simulink model "RightInvariant_EKF"  (R2016b)
settings: Solver=FixedStepDiscrete  StartTime=0.0  StopTime=inf  RelTol=1e-3  EnableMultiTasking=on
InitFcn:
  | realTimeInitFcn;
  | StateEst_ini
undefined symbols (not defined in the file or in its folder): CassieParameters
libraries: StateEstimation_lib x1
settings Model: SimulationMode=external  TunableVars=B2_lpf_velocity_IMU,c_Kd,c_Kd_abduction,c_Kd_abduction_stand,c_Kd_knee,c_Kd_lateral_stand,c_Kd_pitch,c_Kd_roll,c_Kd_rotation,c_Kd_thigh,c_Kd_toe,c_Kd_toe_stand,c_Kfl_d,c_Kfl_p,c_Kfs_d,c_Kfs_p,c_Kp,c_Kp_abduction,c_Kp_abduction_stand,c_Kp_knee,c_Kp_lateral_stand,c_Kp_pitch,c_Kp_roll,c_Kp_rotation,c_Kp_thigh,c_Kp_toe,c_Kp_toe_stand,c_Kt_d,c_abduction_inward_gain,c_damping_gain,c_damping_threshold,c_fil_para,c_fil_para_x,c_fil_para_y,c_final_abduction,c_final_st_abduction,c_final_sw_LL_ext,c_final_sw_abduction,c_h_LL_cp,c_joint_filter_choice,c_lateral_offset,c_lateral_offset_default,c_lateral_velocity_weight,c_pre_final_sw_abduction,c_sagittal_offset,c_sagittal_offset_default,c_shift_distance,c_shift_time,c_stance_thre_lb,c_stance_thre_ub,c_stand_offset_default,c_standing_switch_time,c_test_frequency,c_test_joint,c_toe_tilt_angle,c_use_calib_spring,c_velocity_toe_tune  TunableVarsStorageClass=Auto,Auto,Auto,Auto,Auto,Auto,Auto,Auto,Auto,Auto,Auto,Auto,Auto,Auto,Auto,Auto,Auto,Auto,Auto,Auto,Auto,Auto,Auto,Auto,Auto,Auto,Auto,Auto,Auto,Auto,Auto,Auto,Auto,Auto,Auto,Auto,Auto,Auto,Auto,Auto,Auto,Auto,Auto,Auto,Auto,Auto,Auto,Auto,Auto,Auto,Auto,Auto,Auto,Auto,Auto,Auto,Auto  TunableVarsTypeQualifier=,,,,,,,,,,,,,,,,,,,,,,,,,,,,,,,,,,,,,,,,,,,,,,,,,,,,,,,,  Creator=robot  LastModifiedBy=Ross Hartley
settings SolverCC: EnableConcurrentExecution=on  ConcurrentTasks=on
settings DataIOCC: SaveFormat=Array  SaveOutput=off  SignalLogging=off  DSMLogging=off  VisualizeSimOutput=off  SaveTime=off
settings OptimizationCC: OptimizeBlockIOStorage=off  BufferReuse=off  GlobalBufferReuse=off  ExpressionFolding=off  LocalBlockOutputs=off  LifeSpan=inf  SimCompilerOptimization=on  AccelVerboseBuild=on
settings DebuggingCC: AllowSymbolicDim=off  SFUnexpectedBacktrackingDiag=warning  SFNoUnconditionalDefaultTransitionDiag=warning  SFExecutionAtInitializationDiag=none
settings HardwareCC: ProdBitPerPointer=32  ProdBitPerSizeT=32  ProdBitPerPtrDiffT=32  ProdLargestAtomicFloat=None  ProdWordSize=32  ProdLongLongMode=on  ProdHWDeviceType=Generic->32-bit x86 compatible
settings ModelReferenceCC: EnableParallelModelReferenceBuilds=on  ParallelModelReferenceMATLABWorkerInit=Copy Base Workspace  ModelReferenceNumInstancesAllowed=Single  PropagateSignalLabelsOutOfModel=off
settings SFSimCC: SFSimEcho=off
settings SFSimCC: SimUserSources=|
  | p_RightToeBottom_src.c
  | p_LeftToeBottom_src.c
  | J_RightToeBottom_src.c
  | J_LeftToeBottom_src.c
  | p_VectorNav_to_RightToeBottom_src.c
  | p_VectorNav_to_LeftToeBottom_src.c
  | J_VectorNav_to_RightToeBottom_src.c
  | J_VectorNav_to_LeftToeBottom_src.c
  | p_VectorNav_to_Pelvis_src.c
  | R_VectorNav_to_Pelvis_src.c
  | J_VectorNav_to_Pelvis_src.c
settings SFSimCC: SimUserIncludeDirs=|
  | ..\..\..\..\Cassie_Model\gen\kin\src
  | ..\..\..\..\Cassie_Model\gen\dyn\src
settings RTWCC: SystemTargetFile=slrt.tlc  TLCOptions=-axPCMaxOverloads=1000000000 -axPCMaxOverloadLen=1000000000  TemplateMakefile=slrt_default_tmf  Description=Simulink Real-Time  RTWUseSimCustomCode=on  CodeExecutionProfiling=on  RTWCompilerOptimization=on
settings RTWCC: CustomInclude=|
  | ..\..\..\..\Cassie_Model\gen\kin\src
  | ..\..\..\..\Cassie_Model\gen\dyn\src
settings RTWCC: CustomSource=|
  | p_RightToeBottom_src.c
  | p_LeftToeBottom_src.c
  | J_RightToeBottom_src.c
  | J_LeftToeBottom_src.c
  | p_VectorNav_to_RightToeBottom_src.c
  | p_VectorNav_to_LeftToeBottom_src.c
  | J_VectorNav_to_RightToeBottom_src.c
  | J_VectorNav_to_LeftToeBottom_src.c
  | p_VectorNav_to_Pelvis_src.c
  | R_VectorNav_to_Pelvis_src.c
  | J_VectorNav_to_Pelvis_src.c
settings CodeAppCC: GenerateComments=off  MaxIdLength=128  SimulinkBlockComments=off
settings SimulinkRealTimeCC: xPCRL32EventNumber=5000 * 50  xPCisDownloadable=off
settings ConfigComp: CovMetricSettings=dw  CovHtmlReporting=on  CovSaveCumulativeToWorkspaceVar=on  CovSaveSingleToWorkspaceVar=on  CovExternalEMLEnable=off

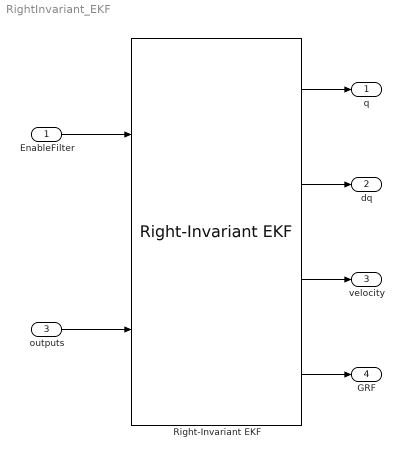
== system RightInvariant_EKF ==
  EnableFilter : Inport  OutDataTypeStr=double  PortDimensions=[1 1]  SampleTime=CassieParameters.etherCatSampleTime  BusOutputAsStruct=on
  outputs : Inport  Port=3  OutDataTypeStr=Bus: cassieOutputsBus  PortDimensions=[1 1]  SampleTime=CassieParameters.etherCatSampleTime  BusOutputAsStruct=on
  Right-Invariant EKF : StateEstimation_lib/Right-Invariant EKF
  q : Outport
  dq : Outport  Port=2
  velocity : Outport  Port=3
  GRF : Outport  Port=4
  wires:
  outputs/1 -> Right-Invariant EKF/2
  EnableFilter/1 -> Right-Invariant EKF/1
  Right-Invariant EKF/1 -> q/1
  Right-Invariant EKF/2 -> dq/1
  Right-Invariant EKF/3 -> velocity/1
  Right-Invariant EKF/4 -> GRF/1
